simulink model "TV_full_sim_V23"  (R2023b)
settings: Solver=FixedStepAuto  StartTime=0.0  StopTime=t_end  FixedStep=ts  RelTol=1e-3
undefined symbols (not defined in the file): a, b, Cf, DGain, Fz_f_static, Fz_r_static, g, h, IGain, Iz, L, load_, m, mu, Mz_dTm_convertion, N_to_lb, NGain, PGain, r_0, vx_vector, vy_0, WT_left, WT_right
libraries: simulink x3, slpidlib x1
settings Model: Creator=savchenko.6  LastModifiedBy=savchenko.6
settings DataIOCC: ReturnWorkspaceOutputs=off

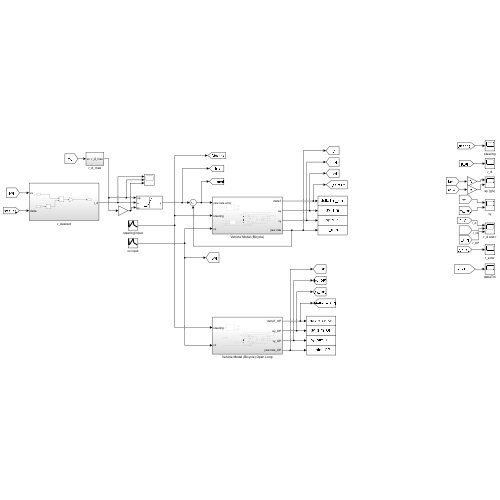
[thumbnail: Simulink's stored preview of the top-level diagram]
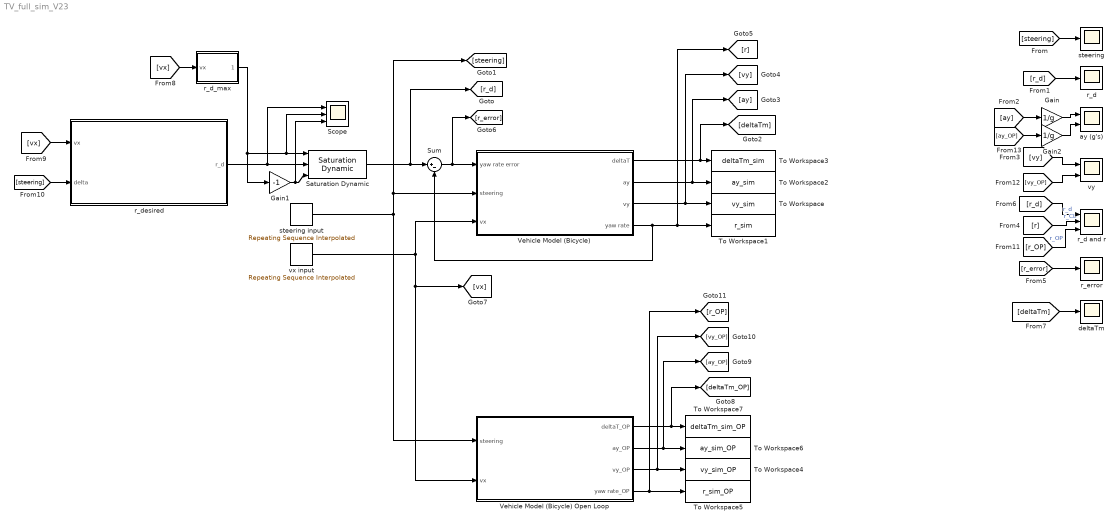
== system TV_full_sim_V23 ==
  Gain : Gain  Gain=1/g
  Gain1 : Gain  Gain=-1
  Gain2 : Gain  Gain=1/g
  Saturation Dynamic : simulink/Discontinuities/Saturation Dynamic  OutMin=[]  OutMax=[]  OutDataTypeStr=Inherit: Same as second input  OutDataType=fixdt(1, 16)  OutScaling=2^-10  RndMeth=Round  DoSatur=off
  Scope : Scope  NumInputPorts=3
  Sum : Sum  Inputs=|+-
  To Workspace : ToWorkspace  VariableName=vy_sim  SampleTime=-1
  To Workspace1 : ToWorkspace  VariableName=r_sim  SampleTime=-1
  To Workspace2 : ToWorkspace  VariableName=ay_sim  SampleTime=-1
  To Workspace3 : ToWorkspace  VariableName=deltaTm_sim  SampleTime=-1
  To Workspace4 : ToWorkspace  VariableName=vy_sim_OP  SampleTime=-1
  To Workspace5 : ToWorkspace  VariableName=r_sim_OP  SampleTime=-1
  To Workspace6 : ToWorkspace  VariableName=ay_sim_OP  SampleTime=-1
  To Workspace7 : ToWorkspace  VariableName=deltaTm_sim_OP  SampleTime=-1
  Vehicle Model (Bicycle) : Subsystem
  Vehicle Model (Bicycle) Open Loop : Subsystem
  ay (g's) : Scope  NumInputPorts=2
  deltaTm : Scope
  r_d : Scope
  r_d and r : Scope  NumInputPorts=3
  r_d_max : Subsystem
  r_desired : Subsystem
  r_error : Scope
  steering : Scope
  steering input : simulink/Sources/Repeating Sequence Interpolated  OutValues=delta  TimeValues=time  LookUpMeth=Interpolation-Use End Values  tsamp=ts  OutMin=[]  OutMax=[]  OutDataTypeStr=double  OutputDataTypeScalingMode=double  OutDataType=fixdt(0,8)  OutScaling=2^-10
  vx input : simulink/Sources/Repeating Sequence Interpolated  OutValues=vx_drive  TimeValues=time  LookUpMeth=Interpolation-Use End Values  tsamp=ts  OutMin=[]  OutMax=[]  OutDataTypeStr=double  OutputDataTypeScalingMode=double  OutDataType=fixdt(0,8)  OutScaling=2^-10
  vy : Scope  NumInputPorts=2
  wires:
  Sum/1 -> [r_error], Vehicle Model (Bicycle)/1(yaw rate error)
  Vehicle Model (Bicycle)/2(ay) -> [ay], To Workspace2/1
  Vehicle Model (Bicycle)/3(vy) -> [vy], To Workspace/1
  Vehicle Model (Bicycle)/4(yaw rate) -> To Workspace1/1, [r], Sum/2
  Vehicle Model (Bicycle)/1(deltaT) -> [deltaTm], To Workspace3/1
  steering input/1 -> [steering], Vehicle Model (Bicycle)/2(steering), Vehicle Model (Bicycle) Open Loop/1(steering)
  [steering] -> steering/1
  [r_d] -> r_d/1
  [ay] -> Gain/1
  [vy] -> vy/1
  [r] -> r_d and r/2  "r_CL"
  [r_error] -> r_error/1
  [r_d] -> r_d and r/1  "r_d"
  vx input/1 -> Vehicle Model (Bicycle) Open Loop/2(vx), [vx], Vehicle Model (Bicycle)/3(vx)
  [deltaTm] -> deltaTm/1
  Gain/1 -> ay (g's)/1
  Saturation Dynamic/1 -> [r_d], Sum/1
  r_d_max/1(r_d_max) -> Scope/2, Saturation Dynamic/1, Gain1/1
  [vx] -> r_d_max/1(vx)
  Gain1/1 -> Scope/3, Saturation Dynamic/3
  [vx] -> r_desired/1(vx)
  [steering] -> r_desired/2(delta)
  r_desired/1(r_d) -> Scope/1, Saturation Dynamic/2
  Vehicle Model (Bicycle) Open Loop/1(deltaT_OP) -> [deltaTm_OP], To Workspace7/1
  Vehicle Model (Bicycle) Open Loop/4(yaw rate_OP) -> [r_OP], To Workspace5/1
  Vehicle Model (Bicycle) Open Loop/2(ay_OP) -> [ay_OP], To Workspace6/1
  Vehicle Model (Bicycle) Open Loop/3(vy_OP) -> [vy_OP], To Workspace4/1
  [r_OP] -> r_d and r/3  "r_OP"
  [vy_OP] -> vy/2
  [ay_OP] -> Gain2/1
  Gain2/1 -> ay (g's)/2

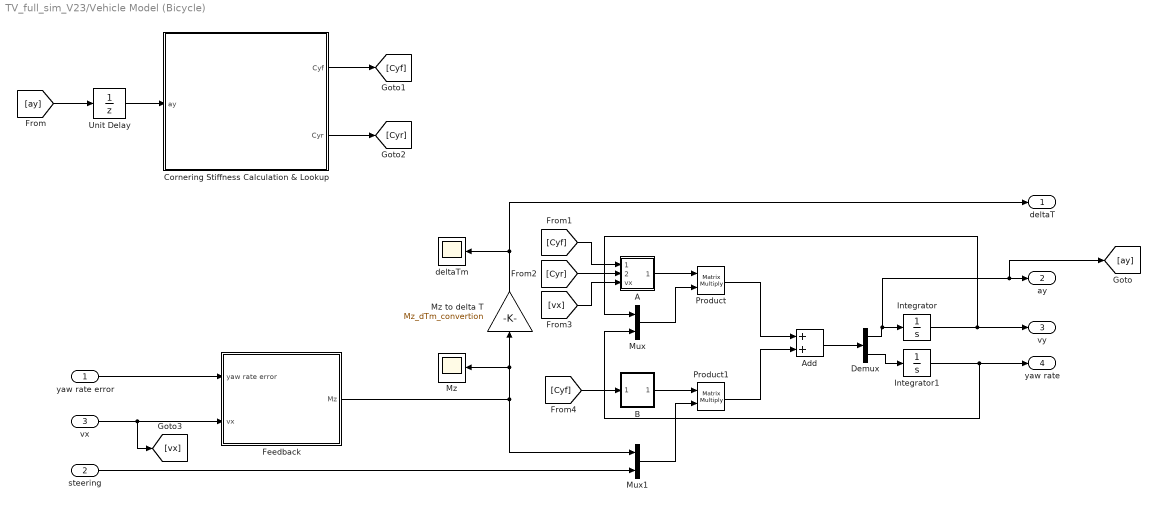
== system TV_full_sim_V23/Vehicle Model (Bicycle) ==
  yaw rate error : Inport
  steering : Inport  Port=2
  vx : Inport  Port=3
  A : Subsystem
  Add : Sum
  B : Subsystem
  Cornering Stiffness Calculation & Lookup : Subsystem
  Demux : Demux  Outputs=2
  Feedback : Subsystem
  Integrator : Integrator  InitialCondition=vy_0
  Integrator1 : Integrator  InitialCondition=r_0
  Mux : Mux  Inputs=2
  Mux1 : Mux  Inputs=2
  Mz : Scope
  Mz to delta T : Gain  Gain=Mz_dTm_convertion
  Product : Product  Multiplication=Matrix(*)
  Product1 : Product  Multiplication=Matrix(*)
  Unit Delay : UnitDelay  SampleTime=-1  HasFrameUpgradeWarning=on
  deltaTm : Scope
  deltaT : Outport
  ay : Outport  Port=2
  vy : Outport  Port=3
  yaw rate : Outport  Port=4
  wires:
  Integrator1/1 -> yaw rate/1, Mux/2
  Add/1 -> Demux/1
  Mz to delta T/1 -> deltaT/1, deltaTm/1
  Mux1/1 -> Product1/2
  Mux/1 -> Product/2
  Product/1 -> Add/1
  Demux/1 -> [ay], ay/1, Integrator/1
  Product1/1 -> Add/2
  Demux/2 -> Integrator1/1
  steering/1 -> Mux1/2
  Integrator/1 -> Mux/1, vy/1
  Feedback/1(Mz) -> Mux1/1, Mz/1, Mz to delta T/1
  yaw rate error/1 -> Feedback/1(yaw rate error)
  vx/1 -> [vx], Feedback/2(vx)
  [ay] -> Unit Delay/1
  Cornering Stiffness Calculation & Lookup/2(Cyr) -> [Cyr]
  [Cyf] -> A/1(Cyf)
  [Cyr] -> A/2(Cyr)
  [vx] -> A/3(vx)
  [Cyf] -> B/1(Cyf)
  Unit Delay/1 -> Cornering Stiffness Calculation & Lookup/1(ay)
  Cornering Stiffness Calculation & Lookup/1(Cyf) -> [Cyf]
  B/1(Out1) -> Product1/1
  A/1(Out1) -> Product/1

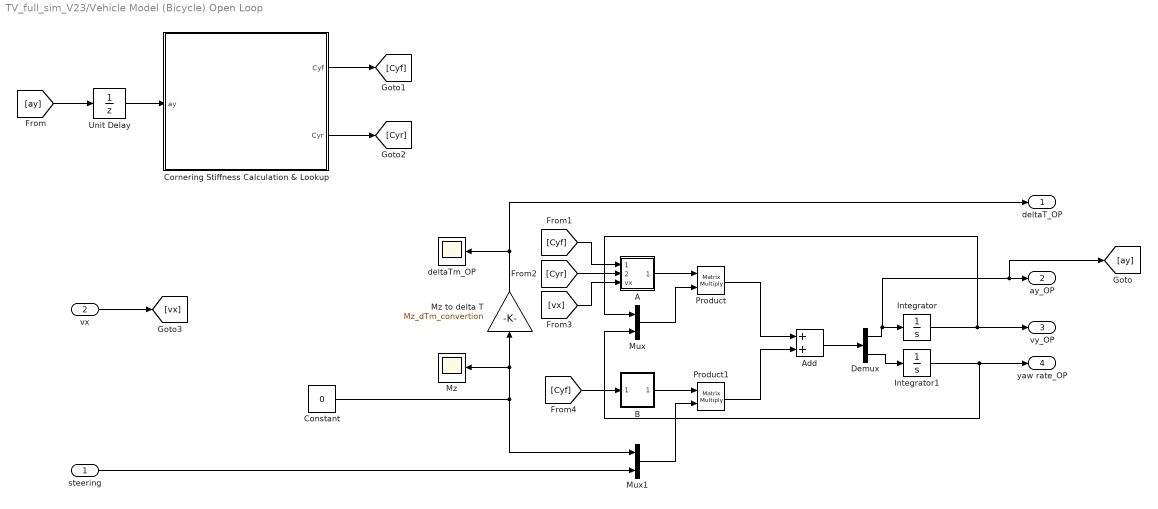
== system TV_full_sim_V23/Vehicle Model (Bicycle) Open Loop ==
  steering : Inport
  vx : Inport  Port=2
  A : Subsystem
  Add : Sum
  B : Subsystem
  Constant : Constant  Value=0
  Cornering Stiffness Calculation & Lookup : Subsystem
  Demux : Demux  Outputs=2
  Integrator : Integrator  InitialCondition=vy_0
  Integrator1 : Integrator  InitialCondition=r_0
  Mux : Mux  Inputs=2
  Mux1 : Mux  Inputs=2
  Mz : Scope
  Mz to delta T : Gain  Gain=Mz_dTm_convertion
  Product : Product  Multiplication=Matrix(*)
  Product1 : Product  Multiplication=Matrix(*)
  Unit Delay : UnitDelay  SampleTime=-1  HasFrameUpgradeWarning=on
  deltaTm_OP : Scope
  deltaT_OP : Outport
  ay_OP : Outport  Port=2
  vy_OP : Outport  Port=3
  yaw rate_OP : Outport  Port=4
  wires:
  Integrator1/1 -> yaw rate_OP/1, Mux/2
  Add/1 -> Demux/1
  Mz to delta T/1 -> deltaT_OP/1, deltaTm_OP/1
  Mux1/1 -> Product1/2
  Mux/1 -> Product/2
  Product/1 -> Add/1
  Demux/1 -> [ay], ay_OP/1, Integrator/1
  Product1/1 -> Add/2
  Demux/2 -> Integrator1/1
  steering/1 -> Mux1/2
  Integrator/1 -> Mux/1, vy_OP/1
  Constant/1 -> Mux1/1, Mz/1, Mz to delta T/1
  [ay] -> Unit Delay/1
  Cornering Stiffness Calculation & Lookup/2(Cyr) -> [Cyr]
  [Cyf] -> A/1(Cyf)
  [Cyr] -> A/2(Cyr)
  [vx] -> A/3(vx)
  [Cyf] -> B/1(Cyf)
  Unit Delay/1 -> Cornering Stiffness Calculation & Lookup/1(ay)
  Cornering Stiffness Calculation & Lookup/1(Cyf) -> [Cyf]
  B/1(Out1) -> Product1/1
  A/1(Out1) -> Product/1
  vx/1 -> [vx]

== system TV_full_sim_V23/r_d_max ==
  vx : Inport
  Constant : Constant  Value=0.85*mu*g/(1+(h/t))
  Divide : Product  Inputs=*/
  Saturation : Saturate  UpperLimit=1000000  LowerLimit=0.01
  r_d_max : Outport
  wires:
  Constant/1 -> Divide/1
  vx/1 -> Saturation/1
  Saturation/1 -> Divide/2
  Divide/1 -> r_d_max/1

== system TV_full_sim_V23/r_desired ==
  vx : Inport
  delta : Inport  Port=2
  Gain : Gain  Gain=1/L
  Product : Product
  Tan : Trigonometry  Operator=tan
  r_d : Outport
  wires:
  delta/1 -> Tan/1
  vx/1 -> Product/1
  Tan/1 -> Product/2
  Product/1 -> Gain/1
  Gain/1 -> r_d/1

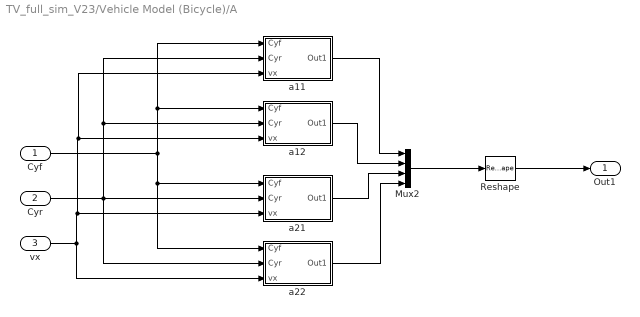
== system TV_full_sim_V23/Vehicle Model (Bicycle)/A ==
  Cyf : Inport
  Cyr : Inport  Port=2
  vx : Inport  Port=3
  Mux2 : Mux
  Reshape : Reshape  OutputDimensionality=Customize  OutputDimensions=[2,2]
  a11 : Subsystem
  a12 : Subsystem
  a21 : Subsystem
  a22 : Subsystem
  Out1 : Outport
  wires:
  a12/1(Out1) -> Mux2/2
  a11/1(Out1) -> Mux2/1
  Reshape/1 -> Out1/1
  a21/1(Out1) -> Mux2/3
  Mux2/1 -> Reshape/1
  a22/1(Out1) -> Mux2/4
  Cyf/1 -> a12/1(Cyf), a11/1(Cyf), a22/1(Cyf), a21/1(Cyf)
  Cyr/1 -> a22/2(Cyr), a21/2(Cyr), a12/2(Cyr), a11/2(Cyr)
  vx/1 -> a22/3(vx), a11/3(vx), a12/3(vx), a21/3(vx)

== system TV_full_sim_V23/Vehicle Model (Bicycle)/B ==
  Cyf : Inport
  Constant : Constant  Value=0
  Constant2 : Constant  Value=1/Iz
  Gain : Gain  Gain=1/m
  Gain1 : Gain  Gain=a/Iz
  Mux2 : Mux
  Reshape : Reshape  OutputDimensionality=Customize  OutputDimensions=[2,2]
  Out1 : Outport
  wires:
  Constant2/1 -> Mux2/3
  Gain/1 -> Mux2/2
  Cyf/1 -> Gain1/1, Gain/1
  Gain1/1 -> Mux2/4
  Reshape/1 -> Out1/1
  Constant/1 -> Mux2/1
  Mux2/1 -> Reshape/1

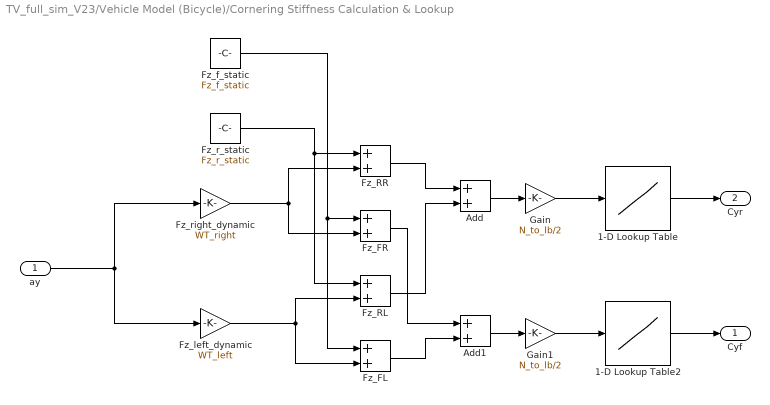
== system TV_full_sim_V23/Vehicle Model (Bicycle)/Cornering Stiffness Calculation & Lookup ==
  ay : Inport
  1-D Lookup Table : Lookup_n-D  NumberOfTableDimensions=1  LookupTableObject=''  BreakpointsForDimension1=load_  BreakpointsForDimension1FirstPoint=10  BreakpointsForDimension2FirstPoint=10  BreakpointsForDimension1Spacing=12  BreakpointsForDimension2Spacing=12  IndexSearchMethod=Evenly spaced points  Table=Cf  RemoveProtectionInput=on  InternalRulePriority=Speed  RndMeth=Simplest  SaturateOnIntegerOverflow=on
  1-D Lookup Table2 : Lookup_n-D  NumberOfTableDimensions=1  LookupTableObject=''  BreakpointsForDimension1=load_  BreakpointsForDimension1FirstPoint=10  BreakpointsForDimension2FirstPoint=10  BreakpointsForDimension1Spacing=12  BreakpointsForDimension2Spacing=12  IndexSearchMethod=Evenly spaced points  Table=Cf  RemoveProtectionInput=on  InternalRulePriority=Speed  RndMeth=Simplest  SaturateOnIntegerOverflow=on
  Add : Sum
  Add1 : Sum
  Fz_FL : Sum
  Fz_FR : Sum
  Fz_RL : Sum
  Fz_RR : Sum
  Fz_f_static : Constant  Value=Fz_f_static
  Fz_left_dynamic : Gain  Gain=WT_left
  Fz_r_static : Constant  Value=Fz_r_static
  Fz_right_dynamic : Gain  Gain=WT_right
  Gain : Gain  Gain=N_to_lb/2
  Gain1 : Gain  Gain=N_to_lb/2
  Cyf : Outport
  Cyr : Outport  Port=2
  wires:
  ay/1 -> Fz_left_dynamic/1, Fz_right_dynamic/1
  Fz_right_dynamic/1 -> Fz_FR/2, Fz_RR/2
  Fz_left_dynamic/1 -> Fz_FL/2, Fz_RL/2
  Fz_f_static/1 -> Fz_FL/1, Fz_FR/1
  Fz_r_static/1 -> Fz_RL/1, Fz_RR/1
  Add/1 -> Gain/1
  Add1/1 -> Gain1/1
  Gain/1 -> 1-D Lookup Table/1
  Gain1/1 -> 1-D Lookup Table2/1
  Fz_RR/1 -> Add/1
  Fz_RL/1 -> Add/2
  Fz_FR/1 -> Add1/1
  Fz_FL/1 -> Add1/2
  1-D Lookup Table/1 -> Cyr/1
  1-D Lookup Table2/1 -> Cyf/1

== system TV_full_sim_V23/Vehicle Model (Bicycle)/Feedback ==
  yaw rate error : Inport
  vx : Inport  Port=2
  D Gains : Lookup_n-D  NumberOfTableDimensions=1  LookupTableObject=''  BreakpointsForDimension1=vx_vector  BreakpointsForDimension1FirstPoint=10  BreakpointsForDimension2FirstPoint=10  BreakpointsForDimension1Spacing=12  BreakpointsForDimension2Spacing=12  IndexSearchMethod=Evenly spaced points  Table=DGain  RemoveProtectionInput=on  InternalRulePriority=Speed  RndMeth=Simplest
  I Gains : Lookup_n-D  NumberOfTableDimensions=1  LookupTableObject=''  BreakpointsForDimension1=vx_vector  BreakpointsForDimension1FirstPoint=10  BreakpointsForDimension2FirstPoint=10  BreakpointsForDimension1Spacing=12  BreakpointsForDimension2Spacing=12  IndexSearchMethod=Evenly spaced points  Table=IGain  RemoveProtectionInput=on  InternalRulePriority=Speed  RndMeth=Simplest
  N Gains : Lookup_n-D  NumberOfTableDimensions=1  LookupTableObject=''  BreakpointsForDimension1=vx_vector  BreakpointsForDimension1FirstPoint=10  BreakpointsForDimension2FirstPoint=10  BreakpointsForDimension1Spacing=12  BreakpointsForDimension2Spacing=12  IndexSearchMethod=Evenly spaced points  Table=NGain  RemoveProtectionInput=on  InternalRulePriority=Speed  RndMeth=Simplest
  P Gains : Lookup_n-D  NumberOfTableDimensions=1  LookupTableObject=''  BreakpointsForDimension1=vx_vector  BreakpointsForDimension1FirstPoint=10  BreakpointsForDimension2FirstPoint=10  BreakpointsForDimension1Spacing=12  BreakpointsForDimension2Spacing=12  IndexSearchMethod=Evenly spaced points  Table=PGain  RemoveProtectionInput=on  InternalRulePriority=Speed  RndMeth=Simplest
  PID Controller : slpidlib/PID Controller  Controller=PID  Form=Parallel  TimeDomain=Continuous-time  UseExternalTs=off  SampleTime=-1  IntegratorMethod=Forward Euler  FilterMethod=Forward Euler  ControllerParametersSource=external  P=122.511124072632  I=58.1909076470783  UseKiTs=off  D=21.7107369694367  N=2  UseFilter=on  TunerSelectOption=Transfer Function Based (PID Tuner App)  InitialConditionSource=internal  InitialConditionForIntegrator=0  InitialConditionForFilter=0  DifferentiatorICPrevScaledInput=0  ExternalReset=none  TrackingMode=off  Kt=1  LimitOutput=off  SatLimitsSource=internal  UpperSaturationLimit=inf  LowerSaturationLimit=-inf  LinearizeAsGain=on  AntiWindupMode=none  Kb=1  LimitIntegrator=off  UpperIntegratorSaturationLimit=inf  LowerIntegratorSaturationLimit=-inf  POutMin=[]  POutMax=[]  IOutMin=[]  IOutMax=[]  DOutMin=[]  DOutMax=[]  NOutMin=[]  NOutMax=[]  SumOutMin=[]  SumOutMax=[]  SaturationOutMin=[]  SaturationOutMax=[]  PParamMin=[]  PParamMax=[]  IParamMin=[]  IParamMax=[]  DParamMin=[]  DParamMax=[]  NParamMin=[]  NParamMax=[]  KbParamMin=[]  KbParamMax=[]  KtParamMin=[]  KtParamMax=[]  KbOutMin=[]  KbOutMax=[]  KtOutMin=[]  KtOutMax=[]  IntegratorOutMin=[]  IntegratorOutMax=[]  FilterOutMin=[]  FilterOutMax=[]  SumI1OutMin=[]  SumI1OutMax=[]  SumI2OutMin=[]  SumI2OutMax=[]  SumI3OutMin=[]  SumI3OutMax=[]  SumI4OutMin=[]  SumI4OutMax=[]  SumDOutMin=[]  SumDOutMax=[]  DifferentiatorOutMin=[]  DifferentiatorOutMax=[]  FilterDiffOutCoefMin=[]  FilterDiffOutCoefMax=[]  ReciprocalOutMin=[]  ReciprocalOutMax=[]  SumDenOutMin=[]  SumDenOutMax=[]  SumNumOutMin=[]  SumNumOutMax=[]  DivideOutMin=[]  DivideOutMax=[]  UdiffTsProdOutMin=[]  UdiffTsProdOutMax=[]  NTsProdOutMin=[]  NTsProdOutMax=[]  UintegralTsProdOutMin=[]  UintegralTsProdOutMax=[]  UngainTsProdOutMin=[]  UngainTsProdOutMax=[]  ClampingZeroOutDataTypeStr=Inherit: Inherit via back propagation  ClampingZeroOutMin=[]  ClampingZeroOutMax=[]  FilterDenConstantOutDataTypeStr=Inherit: Inherit via back propagation  FilterDenConstantOutMin=[]  FilterDenConstantOutMax=[]  PCopyOutDataTypeStr=Inherit: Inherit via back propagation  PCopyOutMin=[]  PCopyOutMax=[]  NCopyOutDataTypeStr=Inherit: Inherit via back propagation  NCopyOutMin=[]  NCopyOutMax=[]  IntegratorContinuousStateAttributes=''  IntegratorStateMustResolveToSignalObject=off  IntegratorRTWStateStorageClass=Auto  FilterContinuousStateAttributes=''  FilterStateMustResolveToSignalObject=off  FilterRTWStateStorageClass=Auto  ParallelPVariant=ExternalParameters  IdealPVariant=Disabled  IVariant=ExternalParameters  DVariant=ExternalParameters  IntegratorVariant=Continuous  SatVariant=Disabled  AWVariant=Passthrough  PCopyVariant=Disabled  TRVariant=Disabled  FdbkBlocksVariant=Forward  IdealPFdbkVariant=Disabled  SatFdbkVariant=Disabled  DerivativeFilterVariant=ContFilter  NVariant=ExternalParameters  NCopyVariant=Disabled  FilterICVariant=InternalICsFilter  IntegratorICVariant=InternalICs  ExternalResetVariant=Disabled  TRSumVariant=Passthrough  SumFdbkVariant=Disabled  SumVariant=Sum_PID  TsampFilterVariant=InternalTs  TsampNgainVariant=Passthrough  TsampIntegralVariant=Disabled_SignalSpec  ExternalSaturationOutDataTypeStr=Inherit: Same as second input
  Mz : Outport
  wires:
  yaw rate error/1 -> PID Controller/1
  PID Controller/1 -> Mz/1
  vx/1 -> N Gains/1, D Gains/1, I Gains/1, P Gains/1
  P Gains/1 -> PID Controller/2
  I Gains/1 -> PID Controller/3
  D Gains/1 -> PID Controller/4
  N Gains/1 -> PID Controller/5

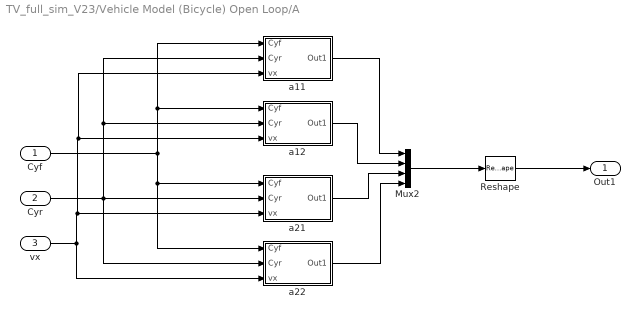
== system TV_full_sim_V23/Vehicle Model (Bicycle) Open Loop/A ==
  Cyf : Inport
  Cyr : Inport  Port=2
  vx : Inport  Port=3
  Mux2 : Mux
  Reshape : Reshape  OutputDimensionality=Customize  OutputDimensions=[2,2]
  a11 : Subsystem
  a12 : Subsystem
  a21 : Subsystem
  a22 : Subsystem
  Out1 : Outport
  wires:
  a12/1(Out1) -> Mux2/2
  a11/1(Out1) -> Mux2/1
  Reshape/1 -> Out1/1
  a21/1(Out1) -> Mux2/3
  Mux2/1 -> Reshape/1
  a22/1(Out1) -> Mux2/4
  Cyf/1 -> a12/1(Cyf), a11/1(Cyf), a22/1(Cyf), a21/1(Cyf)
  Cyr/1 -> a22/2(Cyr), a21/2(Cyr), a12/2(Cyr), a11/2(Cyr)
  vx/1 -> a22/3(vx), a11/3(vx), a12/3(vx), a21/3(vx)

== system TV_full_sim_V23/Vehicle Model (Bicycle) Open Loop/B ==
  Cyf : Inport
  Constant : Constant  Value=0
  Constant2 : Constant  Value=1/Iz
  Gain : Gain  Gain=1/m
  Gain1 : Gain  Gain=a/Iz
  Mux2 : Mux
  Reshape : Reshape  OutputDimensionality=Customize  OutputDimensions=[2,2]
  Out1 : Outport
  wires:
  Constant2/1 -> Mux2/3
  Gain/1 -> Mux2/2
  Cyf/1 -> Gain1/1, Gain/1
  Gain1/1 -> Mux2/4
  Reshape/1 -> Out1/1
  Constant/1 -> Mux2/1
  Mux2/1 -> Reshape/1

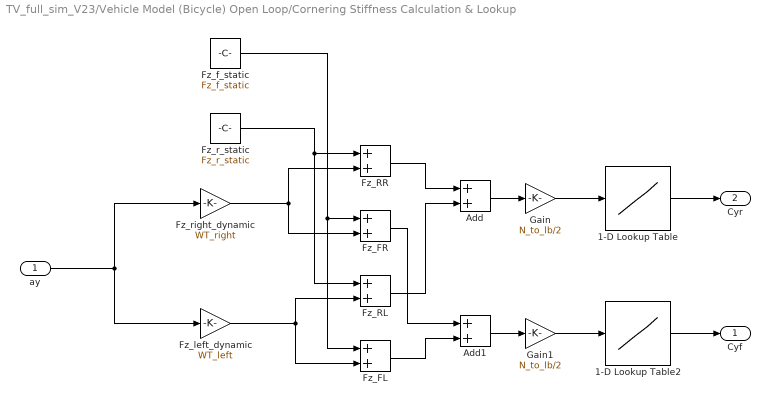
== system TV_full_sim_V23/Vehicle Model (Bicycle) Open Loop/Cornering Stiffness Calculation & Lookup ==
  ay : Inport
  1-D Lookup Table : Lookup_n-D  NumberOfTableDimensions=1  LookupTableObject=''  BreakpointsForDimension1=load_  BreakpointsForDimension1FirstPoint=10  BreakpointsForDimension2FirstPoint=10  BreakpointsForDimension1Spacing=12  BreakpointsForDimension2Spacing=12  IndexSearchMethod=Evenly spaced points  Table=Cf  RemoveProtectionInput=on  InternalRulePriority=Speed  RndMeth=Simplest  SaturateOnIntegerOverflow=on
  1-D Lookup Table2 : Lookup_n-D  NumberOfTableDimensions=1  LookupTableObject=''  BreakpointsForDimension1=load_  BreakpointsForDimension1FirstPoint=10  BreakpointsForDimension2FirstPoint=10  BreakpointsForDimension1Spacing=12  BreakpointsForDimension2Spacing=12  IndexSearchMethod=Evenly spaced points  Table=Cf  RemoveProtectionInput=on  InternalRulePriority=Speed  RndMeth=Simplest  SaturateOnIntegerOverflow=on
  Add : Sum
  Add1 : Sum
  Fz_FL : Sum
  Fz_FR : Sum
  Fz_RL : Sum
  Fz_RR : Sum
  Fz_f_static : Constant  Value=Fz_f_static
  Fz_left_dynamic : Gain  Gain=WT_left
  Fz_r_static : Constant  Value=Fz_r_static
  Fz_right_dynamic : Gain  Gain=WT_right
  Gain : Gain  Gain=N_to_lb/2
  Gain1 : Gain  Gain=N_to_lb/2
  Cyf : Outport
  Cyr : Outport  Port=2
  wires:
  ay/1 -> Fz_left_dynamic/1, Fz_right_dynamic/1
  Fz_right_dynamic/1 -> Fz_FR/2, Fz_RR/2
  Fz_left_dynamic/1 -> Fz_FL/2, Fz_RL/2
  Fz_f_static/1 -> Fz_FL/1, Fz_FR/1
  Fz_r_static/1 -> Fz_RL/1, Fz_RR/1
  Add/1 -> Gain/1
  Add1/1 -> Gain1/1
  Gain/1 -> 1-D Lookup Table/1
  Gain1/1 -> 1-D Lookup Table2/1
  Fz_RR/1 -> Add/1
  Fz_RL/1 -> Add/2
  Fz_FR/1 -> Add1/1
  Fz_FL/1 -> Add1/2
  1-D Lookup Table/1 -> Cyr/1
  1-D Lookup Table2/1 -> Cyf/1

== system TV_full_sim_V23/Vehicle Model (Bicycle)/A/a11 ==
  Cyf : Inport
  Cyr : Inport  Port=2
  vx : Inport  Port=3
  Add1 : Sum
  Divide : Product  Inputs=*/
  Gain : Gain  Gain=-1/m
  Saturation : Saturate  UpperLimit=10000  LowerLimit=0.01
  Out1 : Outport
  wires:
  Cyf/1 -> Add1/1
  Gain/1 -> Divide/1
  Divide/1 -> Out1/1
  Add1/1 -> Gain/1
  vx/1 -> Saturation/1
  Cyr/1 -> Add1/2
  Saturation/1 -> Divide/2

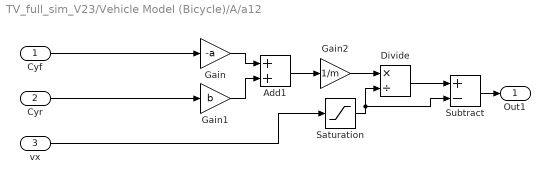
== system TV_full_sim_V23/Vehicle Model (Bicycle)/A/a12 ==
  Cyf : Inport
  Cyr : Inport  Port=2
  vx : Inport  Port=3
  Add1 : Sum
  Divide : Product  Inputs=*/
  Gain : Gain  Gain=-a
  Gain1 : Gain  Gain=b
  Gain2 : Gain  Gain=1/m
  Saturation : Saturate  UpperLimit=10000  LowerLimit=0.01
  Subtract : Sum  Inputs=+-
  Out1 : Outport
  wires:
  Gain/1 -> Add1/1
  Cyr/1 -> Gain1/1
  vx/1 -> Saturation/1
  Gain2/1 -> Divide/1
  Add1/1 -> Gain2/1
  Divide/1 -> Subtract/1
  Gain1/1 -> Add1/2
  Cyf/1 -> Gain/1
  Subtract/1 -> Out1/1
  Saturation/1 -> Subtract/2, Divide/2

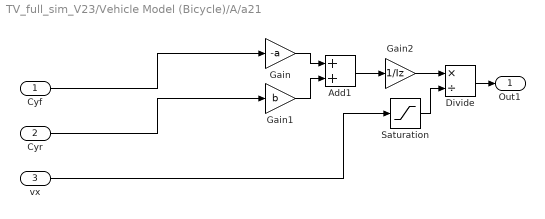
== system TV_full_sim_V23/Vehicle Model (Bicycle)/A/a21 ==
  Cyf : Inport
  Cyr : Inport  Port=2
  vx : Inport  Port=3
  Add1 : Sum
  Divide : Product  Inputs=*/
  Gain : Gain  Gain=-a
  Gain1 : Gain  Gain=b
  Gain2 : Gain  Gain=1/Iz
  Saturation : Saturate  UpperLimit=10000  LowerLimit=0.01
  Out1 : Outport
  wires:
  Cyr/1 -> Gain1/1
  vx/1 -> Saturation/1
  Cyf/1 -> Gain/1
  Gain1/1 -> Add1/2
  Gain2/1 -> Divide/1
  Gain/1 -> Add1/1
  Add1/1 -> Gain2/1
  Divide/1 -> Out1/1
  Saturation/1 -> Divide/2

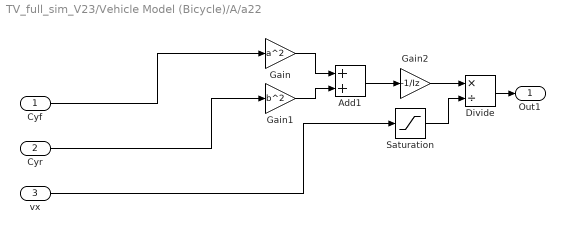
== system TV_full_sim_V23/Vehicle Model (Bicycle)/A/a22 ==
  Cyf : Inport
  Cyr : Inport  Port=2
  vx : Inport  Port=3
  Add1 : Sum
  Divide : Product  Inputs=*/
  Gain : Gain  Gain=a^2
  Gain1 : Gain  Gain=b^2
  Gain2 : Gain  Gain=-1/Iz
  Saturation : Saturate  UpperLimit=10000  LowerLimit=0.01
  Out1 : Outport
  wires:
  Cyr/1 -> Gain1/1
  Gain/1 -> Add1/1
  Divide/1 -> Out1/1
  Add1/1 -> Gain2/1
  Gain1/1 -> Add1/2
  Gain2/1 -> Divide/1
  vx/1 -> Saturation/1
  Cyf/1 -> Gain/1
  Saturation/1 -> Divide/2

== system TV_full_sim_V23/Vehicle Model (Bicycle) Open Loop/A/a11 ==
  Cyf : Inport
  Cyr : Inport  Port=2
  vx : Inport  Port=3
  Add1 : Sum
  Divide : Product  Inputs=*/
  Gain : Gain  Gain=-1/m
  Saturation : Saturate  UpperLimit=10000  LowerLimit=0.01
  Out1 : Outport
  wires:
  Cyf/1 -> Add1/1
  Gain/1 -> Divide/1
  Divide/1 -> Out1/1
  Add1/1 -> Gain/1
  vx/1 -> Saturation/1
  Cyr/1 -> Add1/2
  Saturation/1 -> Divide/2

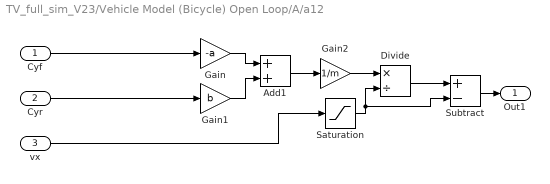
== system TV_full_sim_V23/Vehicle Model (Bicycle) Open Loop/A/a12 ==
  Cyf : Inport
  Cyr : Inport  Port=2
  vx : Inport  Port=3
  Add1 : Sum
  Divide : Product  Inputs=*/
  Gain : Gain  Gain=-a
  Gain1 : Gain  Gain=b
  Gain2 : Gain  Gain=1/m
  Saturation : Saturate  UpperLimit=10000  LowerLimit=0.01
  Subtract : Sum  Inputs=+-
  Out1 : Outport
  wires:
  Gain/1 -> Add1/1
  Cyr/1 -> Gain1/1
  vx/1 -> Saturation/1
  Gain2/1 -> Divide/1
  Add1/1 -> Gain2/1
  Divide/1 -> Subtract/1
  Gain1/1 -> Add1/2
  Cyf/1 -> Gain/1
  Subtract/1 -> Out1/1
  Saturation/1 -> Subtract/2, Divide/2

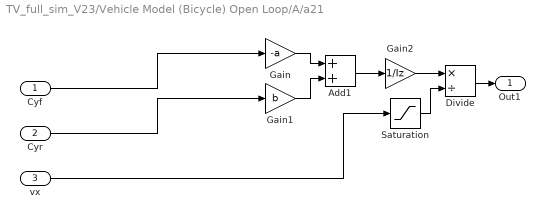
== system TV_full_sim_V23/Vehicle Model (Bicycle) Open Loop/A/a21 ==
  Cyf : Inport
  Cyr : Inport  Port=2
  vx : Inport  Port=3
  Add1 : Sum
  Divide : Product  Inputs=*/
  Gain : Gain  Gain=-a
  Gain1 : Gain  Gain=b
  Gain2 : Gain  Gain=1/Iz
  Saturation : Saturate  UpperLimit=10000  LowerLimit=0.01
  Out1 : Outport
  wires:
  Cyr/1 -> Gain1/1
  vx/1 -> Saturation/1
  Cyf/1 -> Gain/1
  Gain1/1 -> Add1/2
  Gain2/1 -> Divide/1
  Gain/1 -> Add1/1
  Add1/1 -> Gain2/1
  Divide/1 -> Out1/1
  Saturation/1 -> Divide/2

== system TV_full_sim_V23/Vehicle Model (Bicycle) Open Loop/A/a22 ==
  Cyf : Inport
  Cyr : Inport  Port=2
  vx : Inport  Port=3
  Add1 : Sum
  Divide : Product  Inputs=*/
  Gain : Gain  Gain=a^2
  Gain1 : Gain  Gain=b^2
  Gain2 : Gain  Gain=-1/Iz
  Saturation : Saturate  UpperLimit=10000  LowerLimit=0.01
  Out1 : Outport
  wires:
  Cyr/1 -> Gain1/1
  Gain/1 -> Add1/1
  Divide/1 -> Out1/1
  Add1/1 -> Gain2/1
  Gain1/1 -> Add1/2
  Gain2/1 -> Divide/1
  vx/1 -> Saturation/1
  Cyf/1 -> Gain/1
  Saturation/1 -> Divide/2
